simulink model "Twotanks_Model_TCGen"  (R2017b)
settings: Solver=FixedStepAuto  StartTime=0.0  StopTime=simTime  FixedStep=0.1  RelTol=1e-3  EnableMultiTasking=on
model workspace (MAT data in the model file):
  F = [0; 0]
  Global = [3707764736; 2; 1; 1; 1; 1]
  InputSize = 5
  Operation = 'value'
  X = [1.91912110987  0.7189344389; 0.667300428728  0.319032887648; 0.539327875678  0.291550549769; 1.11428719774  0.782058235411; 0.458496889769  0.886118463221]
  cs : Simulink.ConfigSet (value not decoded)
  curPath = '/Users/ceren.gebizli/Desktop/Shiva/QRA-Search/QRA-Search/Problems/SimulinkTesting'
  ext = ''
  generatedFile = '/Users/khouloud.gaaloul/Documents/Projects/SOCRaTeS/socrates/software/scalability/Simulink_Models/Twotanks/Twotanks_Model'
  hws = [3707764736; 2; 1; 1; 1; 1]
  input = [1.91912110987  0.7189344389; 0.667300428728  0.319032887648; 0.539327875678  0.291550549769; 1.11428719774  0.782058235411; 0.458496889769  0.886118463221]
  inputSize = 1
  j = 2
  m = matlab.io.MatFile
  m.Properties = matlab.io.matfile.Properties
  m.Properties.SupportsPartialAccess = 0
  m.Properties.Source = '/Users/khouloud.gaaloul/Documents/Projects/SOCRaTeS/socrates/software/scalability/RQ3/testcases/twotanks_tc_1.mat'
  matfilename = 'twotanks_tc_1.mat'
  model_cs : Simulink.ConfigSet (value not decoded)
  modelpath = '/Users/khouloud.gaaloul/Documents/Projects/SOCRaTeS/socrates/software/scalability/Simulink_Models/Twotanks/'
  name = 'Twotanks_Model'
  nbrInputs = 2
  nbrTimeSteps = 5001
  p = 1
  path = '/Users/khouloud.gaaloul/Documents/Projects/SOCRaTeS/socrates/software/scalability/Simulink_Models/Twotanks'
  pr.model_name = 'Twotanks_Model'
  pr.fc = 5000
  pr.stime = 500
  problem : class16 (value not decoded)
  problems = {'twotanks'}
  tank1_init_height_m = 1.91912110987
  tank2_init_height_m = 0.7189344389
  testcase.signal = [0.0460270741829 0.899426437102]
  timestep = 2
  var.signal = [0.0460270741829 0.899426437102]
values from neighbouring files (symbols this model uses):
  tank1_cross_section_area_m2_in = TC(i).tank1_cross_section_area_m2    [GetWhiteBoxData.m]    (also in MutationTesting.m; TCGeneration.m)
  tank1_pump_flow_rate_m3s_in = TC(i).tank1_pump_flow_rate_m3s    [GetWhiteBoxData.m]    (also in MutationTesting.m; TCGeneration.m)
  tank1_sensor_hi_height_m_in = TC(i).tank1_sensor_hi_height_m    [GetWhiteBoxData.m]    (also in MutationTesting.m; TCGeneration.m)
  tank1_sensor_lo_height_m_in = TC(i).tank1_sensor_lo_height_m    [GetWhiteBoxData.m]    (also in MutationTesting.m; TCGeneration.m)
  tank1_valve_flow_rate_m3s_in = TC(i).tank1_valve_flow_rate_m3s    [GetWhiteBoxData.m]    (also in MutationTesting.m; TCGeneration.m)
  tank2_cross_section_area_m2_in = TC(i).tank2_cross_section_area_m2    [GetWhiteBoxData.m]    (also in MutationTesting.m; TCGeneration.m)
  tank2_e_valve_flow_rate_m3s_in = TC(i).tank2_e_valve_flow_rate_m3s    [GetWhiteBoxData.m]    (also in MutationTesting.m; TCGeneration.m)
  tank2_p_valve_flow_rate_m3s_in = TC(i).tank2_p_valve_flow_rate_m3s    [GetWhiteBoxData.m]    (also in MutationTesting.m; TCGeneration.m)
  tank2_sensor_hi_height_m_in = TC(i).tank2_sensor_hi_height_m    [GetWhiteBoxData.m]    (also in MutationTesting.m; TCGeneration.m)
  tank2_sensor_lo_height_m_in = TC(i).tank2_sensor_lo_height_m    [GetWhiteBoxData.m]    (also in MutationTesting.m; TCGeneration.m)
  tank2_sensor_md_height_m_in = TC(i).tank2_sensor_md_height_m    [GetWhiteBoxData.m]    (also in MutationTesting.m; TCGeneration.m)
libraries: simulink x12
(part 1 of 2)
settings Model: Creator=Kerianne  LastModifiedBy=ainhoa.arruabarrena
settings DataIOCC: ExternalInput=var  LimitDataPoints=on  SaveFormat=StructureWithTime  SignalLoggingSaveFormat=ModelDataLogs  OutputSaveName=varout  LoggingToFile=on
settings OptimizationCC: DefaultParameterBehavior=Inlined  ExpressionDepthLimit=2147483647  LifeSpan=inf
settings DebuggingCC: UnderspecifiedInitializationDetection=Classic  MergeDetectMultiDrivingBlocksExec=none  SolverPrmCheckMsg=warning  MultiTaskDSMMsg=warning  MultiTaskCondExecSysMsg=none  StateNameClashWarn=warning  SFUnexpectedBacktrackingDiag=warning  SFNoUnconditionalDefaultTransitionDiag=warning  SFExecutionAtInitializationDiag=none
settings HardwareCC: ProdBitPerPointer=32  ProdBitPerSizeT=32  ProdBitPerPtrDiffT=32  ProdLargestAtomicFloat=None  ProdIntDivRoundTo=Undefined  ProdEndianess=Unspecified  ProdWordSize=32  ProdHWDeviceType=32-bit Generic
settings ModelReferenceCC: PropagateSignalLabelsOutOfModel=off
settings CodeAppCC: StateflowObjectComments=on
settings GRTTargetCC: TargetLangStandard=C89/C90 (ANSI)  GeneratePreprocessorConditionals=Disable all
settings ConfigComp: CovMetricSettings=dw  CovHtmlReporting=on  CovSaveCumulativeToWorkspaceVar=on  CovSaveSingleToWorkspaceVar=on  CovExternalEMLEnable=off

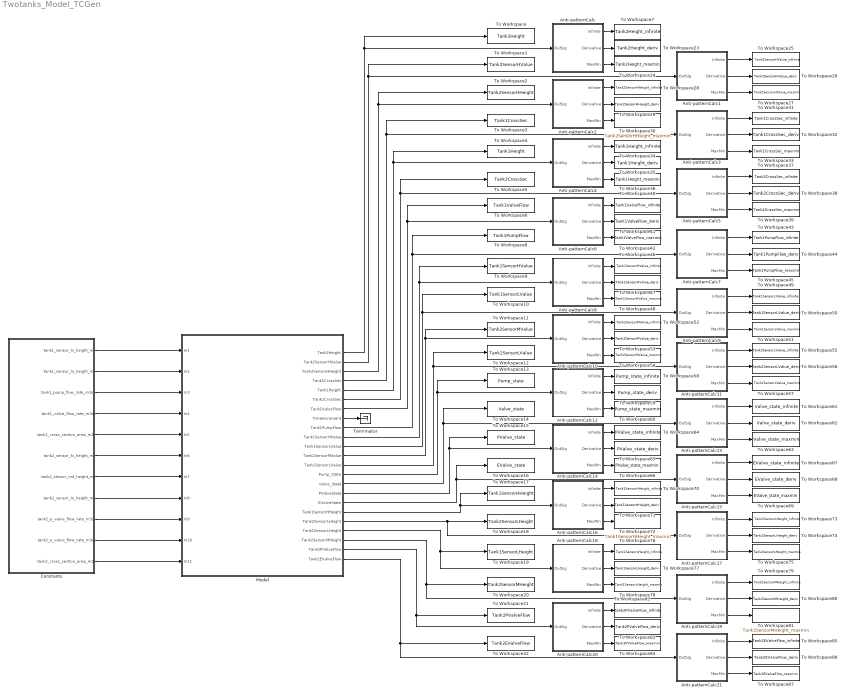
== system Twotanks_Model_TCGen ==
  Anti-patternCalc : Subsystem
  Anti-patternCalc1 : Subsystem
  Anti-patternCalc10 : Subsystem
  Anti-patternCalc11 : Subsystem
  Anti-patternCalc12 : Subsystem
  Anti-patternCalc13 : Subsystem
  Anti-patternCalc14 : Subsystem
  Anti-patternCalc15 : Subsystem
  Anti-patternCalc16 : Subsystem
  Anti-patternCalc17 : Subsystem
  Anti-patternCalc18 : Subsystem
  Anti-patternCalc19 : Subsystem
  Anti-patternCalc2 : Subsystem
  Anti-patternCalc20 : Subsystem
  Anti-patternCalc21 : Subsystem
  Anti-patternCalc3 : Subsystem
  Anti-patternCalc4 : Subsystem
  Anti-patternCalc5 : Subsystem
  Anti-patternCalc6 : Subsystem
  Anti-patternCalc7 : Subsystem
  Anti-patternCalc8 : Subsystem
  Anti-patternCalc9 : Subsystem
  Constants : Subsystem
  Model : Subsystem
  Terminator : Terminator
  To Workspace : ToWorkspace  VariableName=Tank2Height  SampleTime=-1
  To Workspace1 : ToWorkspace  VariableName=Tank2SensorHValue  SampleTime=-1
  To Workspace10 : ToWorkspace  VariableName=Tank1SensorLValue  SampleTime=-1
  To Workspace11 : ToWorkspace  VariableName=Tank2SensorMValue  SampleTime=-1
  To Workspace12 : ToWorkspace  VariableName=Tank2SensorLValue  SampleTime=-1
  To Workspace13 : ToWorkspace  VariableName=Pump_state  SampleTime=-1
  To Workspace14 : ToWorkspace  VariableName=Valve_state  SampleTime=-1
  To Workspace15 : ToWorkspace  VariableName=PValve_state  SampleTime=-1
  To Workspace16 : ToWorkspace  VariableName=EValve_state  SampleTime=-1
  To Workspace17 : ToWorkspace  VariableName=Tank1SensorHHeight  SampleTime=-1
  To Workspace18 : ToWorkspace  VariableName=Tank2SensorLHeight  SampleTime=-1
  To Workspace19 : ToWorkspace  VariableName=Tank1SensorLHeight  SampleTime=-1
  To Workspace2 : ToWorkspace  VariableName=Tank2SensorHHeight  SampleTime=-1
  To Workspace20 : ToWorkspace  VariableName=Tank2SensorMHeight  SampleTime=-1
  To Workspace21 : ToWorkspace  VariableName=Tank2PValveFlow  SampleTime=-1
  To Workspace22 : ToWorkspace  VariableName=Tank2EValveFlow  SampleTime=-1
  To Workspace23 : ToWorkspace  VariableName=Tank2Height_deriv  SampleTime=-1
  To Workspace24 : ToWorkspace  VariableName=Tank2Height_maxmin  SampleTime=-1
  To Workspace25 : ToWorkspace  VariableName=Tank2SensorHValue_infinite  SampleTime=-1
  To Workspace26 : ToWorkspace  VariableName=Tank2SensorHValue_deriv  SampleTime=-1
  To Workspace27 : ToWorkspace  VariableName=Tank2SensorHValue_maxmin  SampleTime=-1
  To Workspace28 : ToWorkspace  VariableName=Tank2SensorHHeight_infinite  SampleTime=-1
  To Workspace29 : ToWorkspace  VariableName=Tank2SensorHHeight_deriv  SampleTime=-1
  To Workspace3 : ToWorkspace  VariableName=Tank1CrossSec  SampleTime=-1
  To Workspace30 : ToWorkspace  VariableName=Tank2SensorHHeight_maxmin  SampleTime=-1
  To Workspace31 : ToWorkspace  VariableName=Tank1CrossSec_infinite  SampleTime=-1
  To Workspace32 : ToWorkspace  VariableName=Tank1CrossSec_deriv  SampleTime=-1
  To Workspace33 : ToWorkspace  VariableName=Tank1CrossSec_maxmin  SampleTime=-1
  To Workspace34 : ToWorkspace  VariableName=Tank1Height_infinite  SampleTime=-1
  To Workspace35 : ToWorkspace  VariableName=Tank1Height_deriv  SampleTime=-1
  To Workspace36 : ToWorkspace  VariableName=Tank1Height_maxmin  SampleTime=-1
  To Workspace37 : ToWorkspace  VariableName=Tank2CrossSec_infinite  SampleTime=-1
  To Workspace38 : ToWorkspace  VariableName=Tank2CrossSec_deriv  SampleTime=-1
  To Workspace39 : ToWorkspace  VariableName=Tank2CrossSec_maxmin  SampleTime=-1
  To Workspace4 : ToWorkspace  VariableName=Tank1Height  SampleTime=-1
  To Workspace40 : ToWorkspace  VariableName=Tank1ValveFlow_infinite  SampleTime=-1
  To Workspace41 : ToWorkspace  VariableName=Tank1ValveFlow_deriv  SampleTime=-1
  To Workspace42 : ToWorkspace  VariableName=Tank1ValveFlow_maxmin  SampleTime=-1
  To Workspace43 : ToWorkspace  VariableName=Tank1PumpFlow_infinite  SampleTime=-1
  To Workspace44 : ToWorkspace  VariableName=Tank1PumpFlow_deriv  SampleTime=-1
  To Workspace45 : ToWorkspace  VariableName=Tank1PumpFlow_maxmin  SampleTime=-1
  To Workspace46 : ToWorkspace  VariableName=Tank1SensorHValue_infinite  SampleTime=-1
  To Workspace47 : ToWorkspace  VariableName=Tank1SensorHValue_deriv  SampleTime=-1
  To Workspace48 : ToWorkspace  VariableName=Tank1SensorHValue_maxmin  SampleTime=-1
  To Workspace49 : ToWorkspace  VariableName=Tank1SensorLValue_infinite  SampleTime=-1
  To Workspace5 : ToWorkspace  VariableName=Tank2CrossSec  SampleTime=-1
  To Workspace50 : ToWorkspace  VariableName=Tank1SensorLValue_deriv  SampleTime=-1
  To Workspace51 : ToWorkspace  VariableName=Tank1SensorLValue_maxmin  SampleTime=-1
  To Workspace52 : ToWorkspace  VariableName=Tank2SensorMValue_infinite  SampleTime=-1
  To Workspace53 : ToWorkspace  VariableName=Tank2SensorMValue_deriv  SampleTime=-1
  To Workspace54 : ToWorkspace  VariableName=Tank2SensorMValue_maxmin  SampleTime=-1
  To Workspace55 : ToWorkspace  VariableName=Tank2SensorLValue_infinite  SampleTime=-1
  To Workspace56 : ToWorkspace  VariableName=Tank2SensorLValue_deriv  SampleTime=-1
  To Workspace57 : ToWorkspace  VariableName=Tank2SensorLValue_maxmin  SampleTime=-1
  To Workspace58 : ToWorkspace  VariableName=Pump_state_infinite  SampleTime=-1
  To Workspace59 : ToWorkspace  VariableName=Pump_state_deriv  SampleTime=-1
  To Workspace6 : ToWorkspace  VariableName=Tank1ValveFlow  SampleTime=-1
  To Workspace60 : ToWorkspace  VariableName=Pump_state_maxmin  SampleTime=-1
  To Workspace61 : ToWorkspace  VariableName=Valve_state_infinite  SampleTime=-1
  To Workspace62 : ToWorkspace  VariableName=Valve_state_deriv  SampleTime=-1
  To Workspace63 : ToWorkspace  VariableName=Valve_state_maxmin  SampleTime=-1
  To Workspace64 : ToWorkspace  VariableName=PValve_state_infinite  SampleTime=-1
  To Workspace65 : ToWorkspace  VariableName=PValve_state_deriv  SampleTime=-1
  To Workspace66 : ToWorkspace  VariableName=PValve_state_maxmin  SampleTime=-1
  To Workspace67 : ToWorkspace  VariableName=EValve_state_infinite  SampleTime=-1
  To Workspace68 : ToWorkspace  VariableName=EValve_state_deriv  SampleTime=-1
  To Workspace69 : ToWorkspace  VariableName=EValve_state_maxmin  SampleTime=-1
  To Workspace7 : ToWorkspace  VariableName=Tank2Height_infinite  SampleTime=-1
  To Workspace70 : ToWorkspace  VariableName=Tank1SensorHHeight_infinite  SampleTime=-1
  To Workspace71 : ToWorkspace  VariableName=Tank1SensorHHeight_deriv  SampleTime=-1
  To Workspace72 : ToWorkspace  VariableName=Tank1SensorHHeight_maxmin  SampleTime=-1
  To Workspace73 : ToWorkspace  VariableName=Tank2SensorLHeight_infinite  SampleTime=-1
  To Workspace74 : ToWorkspace  VariableName=Tank2SensorLHeight_deriv  SampleTime=-1
  To Workspace75 : ToWorkspace  VariableName=Tank2SensorLHeight_maxmin  SampleTime=-1
  To Workspace76 : ToWorkspace  VariableName=Tank1SensorLHeight_infinite  SampleTime=-1
  To Workspace77 : ToWorkspace  VariableName=Tank1SensorLHeight_deriv  SampleTime=-1
  To Workspace78 : ToWorkspace  VariableName=Tank1SensorLHeight_maxmin  SampleTime=-1
  To Workspace79 : ToWorkspace  VariableName=Tank2SensorMHeight_infinite  SampleTime=-1
  To Workspace8 : ToWorkspace  VariableName=Tank1PumpFlow  SampleTime=-1
  To Workspace80 : ToWorkspace  VariableName=Tank2SensorMHeight_deriv  SampleTime=-1
  To Workspace81 : ToWorkspace  VariableName=Tank2SensorMHeight_maxmin  SampleTime=-1
  To Workspace82 : ToWorkspace  VariableName=Tank2PValveFlow_infinite  SampleTime=-1
  To Workspace83 : ToWorkspace  VariableName=Tank2PValveFlow_deriv  SampleTime=-1
  To Workspace84 : ToWorkspace  VariableName=Tank2PValveFlow_maxmin  SampleTime=-1
  To Workspace85 : ToWorkspace  VariableName=Tank2EValveFlow_infinite  SampleTime=-1
  To Workspace86 : ToWorkspace  VariableName=Tank2EValveFlow_deriv  SampleTime=-1
  To Workspace87 : ToWorkspace  VariableName=Tank2EValveFlow_maxmin  SampleTime=-1
  To Workspace9 : ToWorkspace  VariableName=Tank1SensorHValue  SampleTime=-1
  wires:
  Constants/1(tank1_sensor_hi_height_m) -> Model/1(In1)
  Constants/2(tank1_sensor_lo_height_m) -> Model/2(In2)
  Constants/3(tank1_pump_flow_rate_m3s) -> Model/3(In3)
  Constants/4(tank1_valve_flow_rate_m3s) -> Model/4(In4)
  Constants/5(tank1_cross_section_area_m2) -> Model/5(In5)
  Constants/6(tank2_sensor_hi_height_m) -> Model/6(In6)
  Constants/7(tank2_sensor_md_height_m) -> Model/7(In7)
  Constants/8(tank2_sensor_lo_height_m) -> Model/8(In8)
  Constants/9(tank2_p_valve_flow_rate_m3s) -> Model/9(In9)
  Constants/10(tank2_e_valve_flow_rate_m3s) -> Model/10(In10)
  Constants/11(tank2_cross_section_area_m2) -> Model/11(In11)
  Model/1(Tank2Height) -> To Workspace/1, Anti-patternCalc/1(OutSig)
  Model/2(Tank2SensorHValue) -> Anti-patternCalc1/1(OutSig), To Workspace1/1
  Model/3(Tank2SensorHHeight) -> Anti-patternCalc2/1(OutSig), To Workspace2/1
  Model/7(Tank1ValveFlow) -> Anti-patternCalc6/1(OutSig), To Workspace6/1
  Model/8(TimeIncrement) -> Terminator/1
  Model/6(Tank2CrossSec) -> Anti-patternCalc5/1(OutSig), To Workspace5/1
  Model/5(Tank1Height) -> Anti-patternCalc4/1(OutSig), To Workspace4/1
  Model/9(Tank1PumpFlow) -> To Workspace8/1, Anti-patternCalc7/1(OutSig)
  Model/10(Tank1SensorHValue) -> Anti-patternCalc8/1(OutSig), To Workspace9/1
  Model/11(Tank1SensorLValue) -> To Workspace10/1, Anti-patternCalc9/1(OutSig)
  Model/12(Tank2SensorMValue) -> To Workspace11/1, Anti-patternCalc10/1(OutSig)
  Model/13(Tank2SensorLValue) -> Anti-patternCalc11/1(OutSig), To Workspace12/1
  Model/16(PValveState) -> Anti-patternCalc14/1(OutSig), To Workspace15/1
  Model/15(Valve_State) -> Anti-patternCalc13/1(OutSig), To Workspace14/1
  Model/14(Pump_State) -> Anti-patternCalc12/1(OutSig), To Workspace13/1
  Model/19(Tank2SensorLHeight) -> Anti-patternCalc17/1(OutSig), To Workspace18/1
  Model/18(Tank1SensorHHeight) -> Anti-patternCalc16/1(OutSig), To Workspace17/1
  Model/17(EValveState) -> Anti-patternCalc15/1(OutSig), To Workspace16/1
  Model/20(Tank1SensorLHeight) -> Anti-patternCalc18/1(OutSig), To Workspace19/1
  Model/21(Tank2SensorMHeight) -> To Workspace20/1, Anti-patternCalc19/1(OutSig)
  Model/23(Tank2EValveFlow) -> Anti-patternCalc21/1(OutSig), To Workspace22/1
  Model/22(Tank2PValveFlow) -> Anti-patternCalc20/1(OutSig), To Workspace21/1
  Anti-patternCalc/1(Infinite) -> To Workspace7/1
  Anti-patternCalc/2(Derivative) -> To Workspace23/1
  Anti-patternCalc/3(MaxMin) -> To Workspace24/1
  Anti-patternCalc1/1(Infinite) -> To Workspace25/1
  Anti-patternCalc1/3(MaxMin) -> To Workspace27/1
  Anti-patternCalc1/2(Derivative) -> To Workspace26/1
  Anti-patternCalc2/1(Infinite) -> To Workspace28/1
  Anti-patternCalc2/2(Derivative) -> To Workspace29/1
  Anti-patternCalc2/3(MaxMin) -> To Workspace30/1
  Model/4(Tank1CrossSec) -> Anti-patternCalc3/1(OutSig), To Workspace3/1
  Anti-patternCalc3/3(MaxMin) -> To Workspace33/1
  Anti-patternCalc3/2(Derivative) -> To Workspace32/1
  Anti-patternCalc3/1(Infinite) -> To Workspace31/1
  Anti-patternCalc4/1(Infinite) -> To Workspace34/1
  Anti-patternCalc4/2(Derivative) -> To Workspace35/1
  Anti-patternCalc4/3(MaxMin) -> To Workspace36/1
  Anti-patternCalc5/3(MaxMin) -> To Workspace39/1
  Anti-patternCalc5/2(Derivative) -> To Workspace38/1
  Anti-patternCalc5/1(Infinite) -> To Workspace37/1
  Anti-patternCalc6/1(Infinite) -> To Workspace40/1
  Anti-patternCalc6/2(Derivative) -> To Workspace41/1
  Anti-patternCalc6/3(MaxMin) -> To Workspace42/1
  Anti-patternCalc7/1(Infinite) -> To Workspace43/1
  Anti-patternCalc7/3(MaxMin) -> To Workspace45/1
  Anti-patternCalc7/2(Derivative) -> To Workspace44/1
  Anti-patternCalc8/1(Infinite) -> To Workspace46/1
  Anti-patternCalc8/2(Derivative) -> To Workspace47/1
  Anti-patternCalc8/3(MaxMin) -> To Workspace48/1
  Anti-patternCalc9/1(Infinite) -> To Workspace49/1
  Anti-patternCalc9/2(Derivative) -> To Workspace50/1
  Anti-patternCalc9/3(MaxMin) -> To Workspace51/1
  Anti-patternCalc10/1(Infinite) -> To Workspace52/1
  Anti-patternCalc10/2(Derivative) -> To Workspace53/1
  Anti-patternCalc10/3(MaxMin) -> To Workspace54/1
  Anti-patternCalc11/3(MaxMin) -> To Workspace57/1
  Anti-patternCalc11/2(Derivative) -> To Workspace56/1
  Anti-patternCalc11/1(Infinite) -> To Workspace55/1
  Anti-patternCalc12/1(Infinite) -> To Workspace58/1
  Anti-patternCalc12/2(Derivative) -> To Workspace59/1
  Anti-patternCalc12/3(MaxMin) -> To Workspace60/1
  Anti-patternCalc13/1(Infinite) -> To Workspace61/1
  Anti-patternCalc13/2(Derivative) -> To Workspace62/1
  Anti-patternCalc13/3(MaxMin) -> To Workspace63/1
  Anti-patternCalc14/1(Infinite) -> To Workspace64/1
  Anti-patternCalc14/2(Derivative) -> To Workspace65/1
  Anti-patternCalc14/3(MaxMin) -> To Workspace66/1
  Anti-patternCalc15/3(MaxMin) -> To Workspace69/1
  Anti-patternCalc15/2(Derivative) -> To Workspace68/1
  Anti-patternCalc15/1(Infinite) -> To Workspace67/1
  Anti-patternCalc16/1(Infinite) -> To Workspace70/1
  Anti-patternCalc16/2(Derivative) -> To Workspace71/1
  Anti-patternCalc16/3(MaxMin) -> To Workspace72/1
  Anti-patternCalc17/1(Infinite) -> To Workspace73/1
  Anti-patternCalc17/2(Derivative) -> To Workspace74/1
  Anti-patternCalc17/3(MaxMin) -> To Workspace75/1
  Anti-patternCalc18/1(Infinite) -> To Workspace76/1
  Anti-patternCalc18/2(Derivative) -> To Workspace77/1
  Anti-patternCalc18/3(MaxMin) -> To Workspace78/1
  Anti-patternCalc19/1(Infinite) -> To Workspace79/1
  Anti-patternCalc19/3(MaxMin) -> To Workspace81/1
  Anti-patternCalc19/2(Derivative) -> To Workspace80/1
  Anti-patternCalc20/1(Infinite) -> To Workspace82/1
  Anti-patternCalc20/2(Derivative) -> To Workspace83/1
  Anti-patternCalc20/3(MaxMin) -> To Workspace84/1
  Anti-patternCalc21/1(Infinite) -> To Workspace85/1
  Anti-patternCalc21/2(Derivative) -> To Workspace86/1
  Anti-patternCalc21/3(MaxMin) -> To Workspace87/1

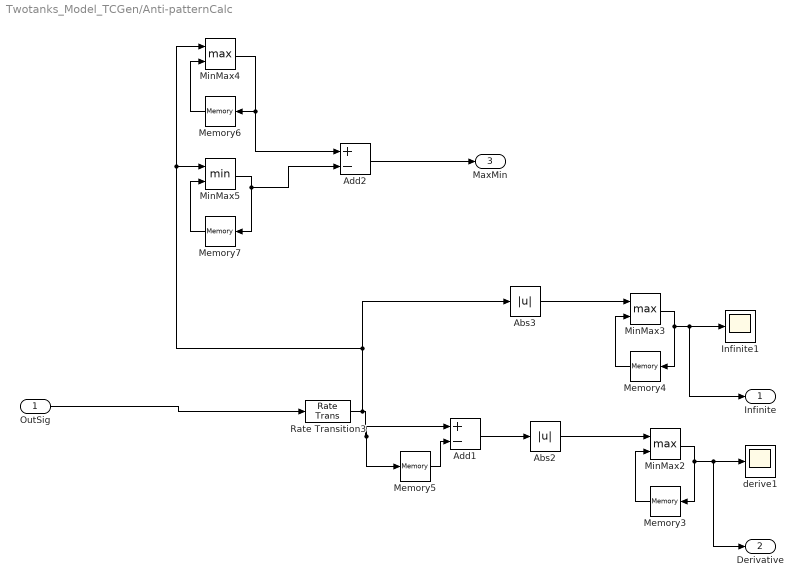
== system Twotanks_Model_TCGen/Anti-patternCalc ==
  OutSig : Inport
  Abs2 : Abs
  Abs3 : Abs
  Add1 : Sum  Inputs=+-
  Add2 : Sum  Inputs=+-
  Infinite1 : Scope
  Memory{3..7} (5 alike) : Memory
  MinMax2 : MinMax  Function=max  Inputs=2
  MinMax3 : MinMax  Function=max  Inputs=2
  MinMax4 : MinMax  Function=max  Inputs=2
  MinMax5 : MinMax  Inputs=2
  Rate Transition3 : RateTransition
  derive1 : Scope
  Infinite : Outport
  Derivative : Outport  Port=2
  MaxMin : Outport  Port=3
  wires:
  MinMax5/1 -> Add2/2, Memory7/1
  Abs2/1 -> MinMax2/1
  Memory4/1 -> MinMax3/2
  Memory3/1 -> MinMax2/2
  MinMax4/1 -> Add2/1, Memory6/1
  Memory7/1 -> MinMax5/2
  Add1/1 -> Abs2/1
  Memory6/1 -> MinMax4/2
  Memory5/1 -> Add1/2
  Rate Transition3/1 -> MinMax4/1, MinMax5/1, Abs3/1, Add1/1, Memory5/1
  Abs3/1 -> MinMax3/1
  MinMax2/1 -> Derivative/1, derive1/1, Memory3/1
  OutSig/1 -> Rate Transition3/1
  MinMax3/1 -> Memory4/1, Infinite/1, Infinite1/1
  Add2/1 -> MaxMin/1

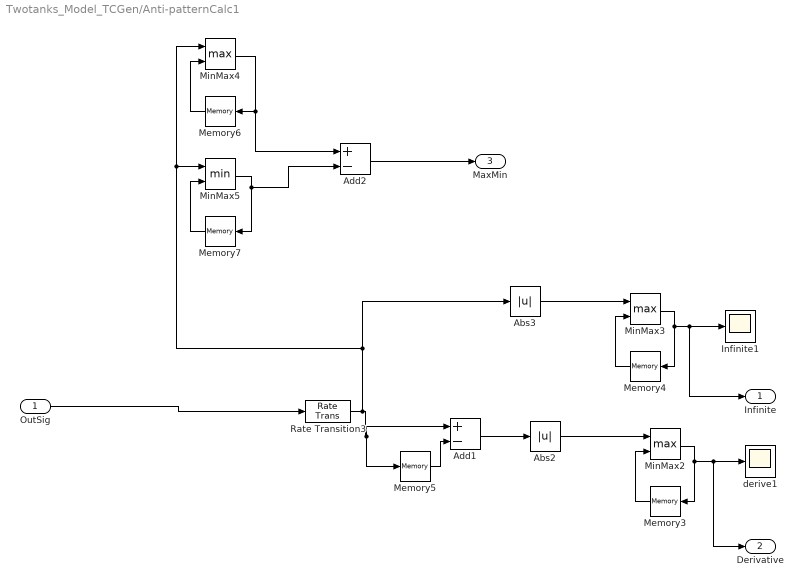
== system Twotanks_Model_TCGen/Anti-patternCalc1 ==
  OutSig : Inport
  Abs2 : Abs
  Abs3 : Abs
  Add1 : Sum  Inputs=+-
  Add2 : Sum  Inputs=+-
  Infinite1 : Scope
  Memory{3..7} (5 alike) : Memory
  MinMax2 : MinMax  Function=max  Inputs=2
  MinMax3 : MinMax  Function=max  Inputs=2
  MinMax4 : MinMax  Function=max  Inputs=2
  MinMax5 : MinMax  Inputs=2
  Rate Transition3 : RateTransition
  derive1 : Scope
  Infinite : Outport
  Derivative : Outport  Port=2
  MaxMin : Outport  Port=3
  wires:
  Add2/1 -> MaxMin/1
  MinMax3/1 -> Infinite1/1, Infinite/1, Memory4/1
  OutSig/1 -> Rate Transition3/1
  MinMax2/1 -> Memory3/1, derive1/1, Derivative/1
  Abs3/1 -> MinMax3/1
  Rate Transition3/1 -> Memory5/1, Add1/1, Abs3/1, MinMax5/1, MinMax4/1
  Memory5/1 -> Add1/2
  Memory6/1 -> MinMax4/2
  Add1/1 -> Abs2/1
  Memory7/1 -> MinMax5/2
  MinMax4/1 -> Memory6/1, Add2/1
  Memory3/1 -> MinMax2/2
  Memory4/1 -> MinMax3/2
  Abs2/1 -> MinMax2/1
  MinMax5/1 -> Memory7/1, Add2/2

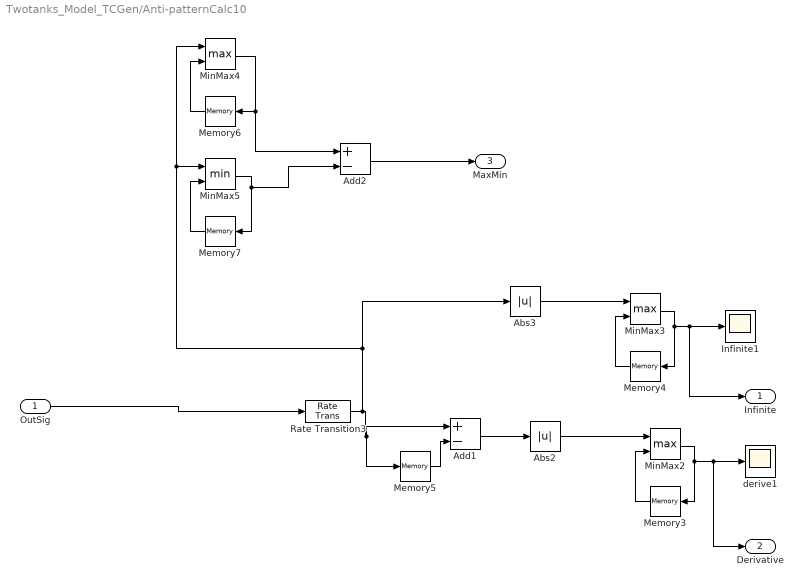
== system Twotanks_Model_TCGen/Anti-patternCalc10 ==
  OutSig : Inport
  Abs2 : Abs
  Abs3 : Abs
  Add1 : Sum  Inputs=+-
  Add2 : Sum  Inputs=+-
  Infinite1 : Scope
  Memory{3..7} (5 alike) : Memory
  MinMax2 : MinMax  Function=max  Inputs=2
  MinMax3 : MinMax  Function=max  Inputs=2
  MinMax4 : MinMax  Function=max  Inputs=2
  MinMax5 : MinMax  Inputs=2
  Rate Transition3 : RateTransition
  derive1 : Scope
  Infinite : Outport
  Derivative : Outport  Port=2
  MaxMin : Outport  Port=3
  wires:
  Add2/1 -> MaxMin/1
  MinMax3/1 -> Infinite1/1, Infinite/1, Memory4/1
  OutSig/1 -> Rate Transition3/1
  MinMax2/1 -> Memory3/1, derive1/1, Derivative/1
  Abs3/1 -> MinMax3/1
  Rate Transition3/1 -> Memory5/1, Add1/1, Abs3/1, MinMax5/1, MinMax4/1
  Memory5/1 -> Add1/2
  Memory6/1 -> MinMax4/2
  Add1/1 -> Abs2/1
  Memory7/1 -> MinMax5/2
  MinMax4/1 -> Memory6/1, Add2/1
  Memory3/1 -> MinMax2/2
  Memory4/1 -> MinMax3/2
  Abs2/1 -> MinMax2/1
  MinMax5/1 -> Memory7/1, Add2/2

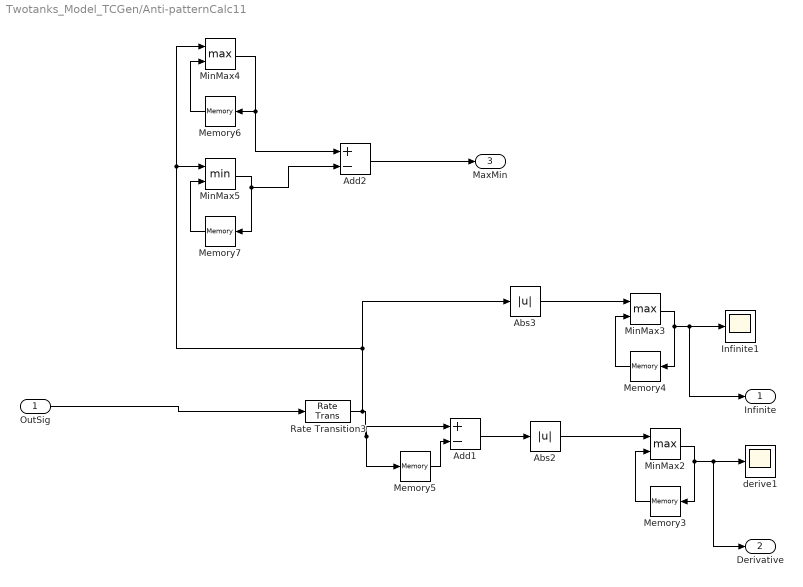
== system Twotanks_Model_TCGen/Anti-patternCalc11 ==
  OutSig : Inport
  Abs2 : Abs
  Abs3 : Abs
  Add1 : Sum  Inputs=+-
  Add2 : Sum  Inputs=+-
  Infinite1 : Scope
  Memory{3..7} (5 alike) : Memory
  MinMax2 : MinMax  Function=max  Inputs=2
  MinMax3 : MinMax  Function=max  Inputs=2
  MinMax4 : MinMax  Function=max  Inputs=2
  MinMax5 : MinMax  Inputs=2
  Rate Transition3 : RateTransition
  derive1 : Scope
  Infinite : Outport
  Derivative : Outport  Port=2
  MaxMin : Outport  Port=3
  wires:
  MinMax5/1 -> Add2/2, Memory7/1
  Abs2/1 -> MinMax2/1
  Memory4/1 -> MinMax3/2
  Memory3/1 -> MinMax2/2
  MinMax4/1 -> Add2/1, Memory6/1
  Memory7/1 -> MinMax5/2
  Add1/1 -> Abs2/1
  Memory6/1 -> MinMax4/2
  Memory5/1 -> Add1/2
  Rate Transition3/1 -> MinMax4/1, MinMax5/1, Abs3/1, Add1/1, Memory5/1
  Abs3/1 -> MinMax3/1
  MinMax2/1 -> Derivative/1, derive1/1, Memory3/1
  OutSig/1 -> Rate Transition3/1
  MinMax3/1 -> Memory4/1, Infinite/1, Infinite1/1
  Add2/1 -> MaxMin/1

== system Twotanks_Model_TCGen/Anti-patternCalc12 ==
  OutSig : Inport
  Abs2 : Abs
  Abs3 : Abs
  Add1 : Sum  Inputs=+-
  Add2 : Sum  Inputs=+-
  Infinite1 : Scope
  Memory{3..7} (5 alike) : Memory
  MinMax2 : MinMax  Function=max  Inputs=2
  MinMax3 : MinMax  Function=max  Inputs=2
  MinMax4 : MinMax  Function=max  Inputs=2
  MinMax5 : MinMax  Inputs=2
  Rate Transition3 : RateTransition
  derive1 : Scope
  Infinite : Outport
  Derivative : Outport  Port=2
  MaxMin : Outport  Port=3
  wires:
  MinMax5/1 -> Add2/2, Memory7/1
  Abs2/1 -> MinMax2/1
  Memory4/1 -> MinMax3/2
  Memory3/1 -> MinMax2/2
  MinMax4/1 -> Add2/1, Memory6/1
  Memory7/1 -> MinMax5/2
  Add1/1 -> Abs2/1
  Memory6/1 -> MinMax4/2
  Memory5/1 -> Add1/2
  Rate Transition3/1 -> MinMax4/1, MinMax5/1, Abs3/1, Add1/1, Memory5/1
  Abs3/1 -> MinMax3/1
  MinMax2/1 -> Derivative/1, derive1/1, Memory3/1
  OutSig/1 -> Rate Transition3/1
  MinMax3/1 -> Memory4/1, Infinite/1, Infinite1/1
  Add2/1 -> MaxMin/1

== system Twotanks_Model_TCGen/Anti-patternCalc13 ==
  OutSig : Inport
  Abs2 : Abs
  Abs3 : Abs
  Add1 : Sum  Inputs=+-
  Add2 : Sum  Inputs=+-
  Infinite1 : Scope
  Memory{3..7} (5 alike) : Memory
  MinMax2 : MinMax  Function=max  Inputs=2
  MinMax3 : MinMax  Function=max  Inputs=2
  MinMax4 : MinMax  Function=max  Inputs=2
  MinMax5 : MinMax  Inputs=2
  Rate Transition3 : RateTransition
  derive1 : Scope
  Infinite : Outport
  Derivative : Outport  Port=2
  MaxMin : Outport  Port=3
  wires:
  Add2/1 -> MaxMin/1
  MinMax3/1 -> Infinite1/1, Infinite/1, Memory4/1
  OutSig/1 -> Rate Transition3/1
  MinMax2/1 -> Memory3/1, derive1/1, Derivative/1
  Abs3/1 -> MinMax3/1
  Rate Transition3/1 -> Memory5/1, Add1/1, Abs3/1, MinMax5/1, MinMax4/1
  Memory5/1 -> Add1/2
  Memory6/1 -> MinMax4/2
  Add1/1 -> Abs2/1
  Memory7/1 -> MinMax5/2
  MinMax4/1 -> Memory6/1, Add2/1
  Memory3/1 -> MinMax2/2
  Memory4/1 -> MinMax3/2
  Abs2/1 -> MinMax2/1
  MinMax5/1 -> Memory7/1, Add2/2

== system Twotanks_Model_TCGen/Anti-patternCalc14 ==
  OutSig : Inport
  Abs2 : Abs
  Abs3 : Abs
  Add1 : Sum  Inputs=+-
  Add2 : Sum  Inputs=+-
  Infinite1 : Scope
  Memory{3..7} (5 alike) : Memory
  MinMax2 : MinMax  Function=max  Inputs=2
  MinMax3 : MinMax  Function=max  Inputs=2
  MinMax4 : MinMax  Function=max  Inputs=2
  MinMax5 : MinMax  Inputs=2
  Rate Transition3 : RateTransition
  derive1 : Scope
  Infinite : Outport
  Derivative : Outport  Port=2
  MaxMin : Outport  Port=3
  wires:
  Add2/1 -> MaxMin/1
  MinMax3/1 -> Infinite1/1, Infinite/1, Memory4/1
  OutSig/1 -> Rate Transition3/1
  MinMax2/1 -> Memory3/1, derive1/1, Derivative/1
  Abs3/1 -> MinMax3/1
  Rate Transition3/1 -> Memory5/1, Add1/1, Abs3/1, MinMax5/1, MinMax4/1
  Memory5/1 -> Add1/2
  Memory6/1 -> MinMax4/2
  Add1/1 -> Abs2/1
  Memory7/1 -> MinMax5/2
  MinMax4/1 -> Memory6/1, Add2/1
  Memory3/1 -> MinMax2/2
  Memory4/1 -> MinMax3/2
  Abs2/1 -> MinMax2/1
  MinMax5/1 -> Memory7/1, Add2/2

== system Twotanks_Model_TCGen/Anti-patternCalc15 ==
  OutSig : Inport
  Abs2 : Abs
  Abs3 : Abs
  Add1 : Sum  Inputs=+-
  Add2 : Sum  Inputs=+-
  Infinite1 : Scope
  Memory{3..7} (5 alike) : Memory
  MinMax2 : MinMax  Function=max  Inputs=2
  MinMax3 : MinMax  Function=max  Inputs=2
  MinMax4 : MinMax  Function=max  Inputs=2
  MinMax5 : MinMax  Inputs=2
  Rate Transition3 : RateTransition
  derive1 : Scope
  Infinite : Outport
  Derivative : Outport  Port=2
  MaxMin : Outport  Port=3
  wires:
  MinMax5/1 -> Add2/2, Memory7/1
  Abs2/1 -> MinMax2/1
  Memory4/1 -> MinMax3/2
  Memory3/1 -> MinMax2/2
  MinMax4/1 -> Add2/1, Memory6/1
  Memory7/1 -> MinMax5/2
  Add1/1 -> Abs2/1
  Memory6/1 -> MinMax4/2
  Memory5/1 -> Add1/2
  Rate Transition3/1 -> MinMax4/1, MinMax5/1, Abs3/1, Add1/1, Memory5/1
  Abs3/1 -> MinMax3/1
  MinMax2/1 -> Derivative/1, derive1/1, Memory3/1
  OutSig/1 -> Rate Transition3/1
  MinMax3/1 -> Memory4/1, Infinite/1, Infinite1/1
  Add2/1 -> MaxMin/1

== system Twotanks_Model_TCGen/Anti-patternCalc16 ==
  OutSig : Inport
  Abs2 : Abs
  Abs3 : Abs
  Add1 : Sum  Inputs=+-
  Add2 : Sum  Inputs=+-
  Infinite1 : Scope
  Memory{3..7} (5 alike) : Memory
  MinMax2 : MinMax  Function=max  Inputs=2
  MinMax3 : MinMax  Function=max  Inputs=2
  MinMax4 : MinMax  Function=max  Inputs=2
  MinMax5 : MinMax  Inputs=2
  Rate Transition3 : RateTransition
  derive1 : Scope
  Infinite : Outport
  Derivative : Outport  Port=2
  MaxMin : Outport  Port=3
  wires:
  MinMax5/1 -> Add2/2, Memory7/1
  Abs2/1 -> MinMax2/1
  Memory4/1 -> MinMax3/2
  Memory3/1 -> MinMax2/2
  MinMax4/1 -> Add2/1, Memory6/1
  Memory7/1 -> MinMax5/2
  Add1/1 -> Abs2/1
  Memory6/1 -> MinMax4/2
  Memory5/1 -> Add1/2
  Rate Transition3/1 -> MinMax4/1, MinMax5/1, Abs3/1, Add1/1, Memory5/1
  Abs3/1 -> MinMax3/1
  MinMax2/1 -> Derivative/1, derive1/1, Memory3/1
  OutSig/1 -> Rate Transition3/1
  MinMax3/1 -> Memory4/1, Infinite/1, Infinite1/1
  Add2/1 -> MaxMin/1

== system Twotanks_Model_TCGen/Anti-patternCalc17 ==
  OutSig : Inport
  Abs2 : Abs
  Abs3 : Abs
  Add1 : Sum  Inputs=+-
  Add2 : Sum  Inputs=+-
  Infinite1 : Scope
  Memory{3..7} (5 alike) : Memory
  MinMax2 : MinMax  Function=max  Inputs=2
  MinMax3 : MinMax  Function=max  Inputs=2
  MinMax4 : MinMax  Function=max  Inputs=2
  MinMax5 : MinMax  Inputs=2
  Rate Transition3 : RateTransition
  derive1 : Scope
  Infinite : Outport
  Derivative : Outport  Port=2
  MaxMin : Outport  Port=3
  wires:
  Add2/1 -> MaxMin/1
  MinMax3/1 -> Infinite1/1, Infinite/1, Memory4/1
  OutSig/1 -> Rate Transition3/1
  MinMax2/1 -> Memory3/1, derive1/1, Derivative/1
  Abs3/1 -> MinMax3/1
  Rate Transition3/1 -> Memory5/1, Add1/1, Abs3/1, MinMax5/1, MinMax4/1
  Memory5/1 -> Add1/2
  Memory6/1 -> MinMax4/2
  Add1/1 -> Abs2/1
  Memory7/1 -> MinMax5/2
  MinMax4/1 -> Memory6/1, Add2/1
  Memory3/1 -> MinMax2/2
  Memory4/1 -> MinMax3/2
  Abs2/1 -> MinMax2/1
  MinMax5/1 -> Memory7/1, Add2/2

== system Twotanks_Model_TCGen/Anti-patternCalc18 ==
  OutSig : Inport
  Abs2 : Abs
  Abs3 : Abs
  Add1 : Sum  Inputs=+-
  Add2 : Sum  Inputs=+-
  Infinite1 : Scope
  Memory{3..7} (5 alike) : Memory
  MinMax2 : MinMax  Function=max  Inputs=2
  MinMax3 : MinMax  Function=max  Inputs=2
  MinMax4 : MinMax  Function=max  Inputs=2
  MinMax5 : MinMax  Inputs=2
  Rate Transition3 : RateTransition
  derive1 : Scope
  Infinite : Outport
  Derivative : Outport  Port=2
  MaxMin : Outport  Port=3
  wires:
  Add2/1 -> MaxMin/1
  MinMax3/1 -> Infinite1/1, Infinite/1, Memory4/1
  OutSig/1 -> Rate Transition3/1
  MinMax2/1 -> Memory3/1, derive1/1, Derivative/1
  Abs3/1 -> MinMax3/1
  Rate Transition3/1 -> Memory5/1, Add1/1, Abs3/1, MinMax5/1, MinMax4/1
  Memory5/1 -> Add1/2
  Memory6/1 -> MinMax4/2
  Add1/1 -> Abs2/1
  Memory7/1 -> MinMax5/2
  MinMax4/1 -> Memory6/1, Add2/1
  Memory3/1 -> MinMax2/2
  Memory4/1 -> MinMax3/2
  Abs2/1 -> MinMax2/1
  MinMax5/1 -> Memory7/1, Add2/2

== system Twotanks_Model_TCGen/Anti-patternCalc19 ==
  OutSig : Inport
  Abs2 : Abs
  Abs3 : Abs
  Add1 : Sum  Inputs=+-
  Add2 : Sum  Inputs=+-
  Infinite1 : Scope
  Memory{3..7} (5 alike) : Memory
  MinMax2 : MinMax  Function=max  Inputs=2
  MinMax3 : MinMax  Function=max  Inputs=2
  MinMax4 : MinMax  Function=max  Inputs=2
  MinMax5 : MinMax  Inputs=2
  Rate Transition3 : RateTransition
  derive1 : Scope
  Infinite : Outport
  Derivative : Outport  Port=2
  MaxMin : Outport  Port=3
  wires:
  MinMax5/1 -> Add2/2, Memory7/1
  Abs2/1 -> MinMax2/1
  Memory4/1 -> MinMax3/2
  Memory3/1 -> MinMax2/2
  MinMax4/1 -> Add2/1, Memory6/1
  Memory7/1 -> MinMax5/2
  Add1/1 -> Abs2/1
  Memory6/1 -> MinMax4/2
  Memory5/1 -> Add1/2
  Rate Transition3/1 -> MinMax4/1, MinMax5/1, Abs3/1, Add1/1, Memory5/1
  Abs3/1 -> MinMax3/1
  MinMax2/1 -> Derivative/1, derive1/1, Memory3/1
  OutSig/1 -> Rate Transition3/1
  MinMax3/1 -> Memory4/1, Infinite/1, Infinite1/1
  Add2/1 -> MaxMin/1

== system Twotanks_Model_TCGen/Anti-patternCalc2 ==
  OutSig : Inport
  Abs2 : Abs
  Abs3 : Abs
  Add1 : Sum  Inputs=+-
  Add2 : Sum  Inputs=+-
  Infinite1 : Scope
  Memory{3..7} (5 alike) : Memory
  MinMax2 : MinMax  Function=max  Inputs=2
  MinMax3 : MinMax  Function=max  Inputs=2
  MinMax4 : MinMax  Function=max  Inputs=2
  MinMax5 : MinMax  Inputs=2
  Rate Transition3 : RateTransition
  derive1 : Scope
  Infinite : Outport
  Derivative : Outport  Port=2
  MaxMin : Outport  Port=3
  wires:
  MinMax5/1 -> Add2/2, Memory7/1
  Abs2/1 -> MinMax2/1
  Memory4/1 -> MinMax3/2
  Memory3/1 -> MinMax2/2
  MinMax4/1 -> Add2/1, Memory6/1
  Memory7/1 -> MinMax5/2
  Add1/1 -> Abs2/1
  Memory6/1 -> MinMax4/2
  Memory5/1 -> Add1/2
  Rate Transition3/1 -> MinMax4/1, MinMax5/1, Abs3/1, Add1/1, Memory5/1
  Abs3/1 -> MinMax3/1
  MinMax2/1 -> Derivative/1, derive1/1, Memory3/1
  OutSig/1 -> Rate Transition3/1
  MinMax3/1 -> Memory4/1, Infinite/1, Infinite1/1
  Add2/1 -> MaxMin/1

== system Twotanks_Model_TCGen/Anti-patternCalc20 ==
  OutSig : Inport
  Abs2 : Abs
  Abs3 : Abs
  Add1 : Sum  Inputs=+-
  Add2 : Sum  Inputs=+-
  Infinite1 : Scope
  Memory{3..7} (5 alike) : Memory
  MinMax2 : MinMax  Function=max  Inputs=2
  MinMax3 : MinMax  Function=max  Inputs=2
  MinMax4 : MinMax  Function=max  Inputs=2
  MinMax5 : MinMax  Inputs=2
  Rate Transition3 : RateTransition
  derive1 : Scope
  Infinite : Outport
  Derivative : Outport  Port=2
  MaxMin : Outport  Port=3
  wires:
  MinMax5/1 -> Add2/2, Memory7/1
  Abs2/1 -> MinMax2/1
  Memory4/1 -> MinMax3/2
  Memory3/1 -> MinMax2/2
  MinMax4/1 -> Add2/1, Memory6/1
  Memory7/1 -> MinMax5/2
  Add1/1 -> Abs2/1
  Memory6/1 -> MinMax4/2
  Memory5/1 -> Add1/2
  Rate Transition3/1 -> MinMax4/1, MinMax5/1, Abs3/1, Add1/1, Memory5/1
  Abs3/1 -> MinMax3/1
  MinMax2/1 -> Derivative/1, derive1/1, Memory3/1
  OutSig/1 -> Rate Transition3/1
  MinMax3/1 -> Memory4/1, Infinite/1, Infinite1/1
  Add2/1 -> MaxMin/1

== system Twotanks_Model_TCGen/Anti-patternCalc21 ==
  OutSig : Inport
  Abs2 : Abs
  Abs3 : Abs
  Add1 : Sum  Inputs=+-
  Add2 : Sum  Inputs=+-
  Infinite1 : Scope
  Memory{3..7} (5 alike) : Memory
  MinMax2 : MinMax  Function=max  Inputs=2
  MinMax3 : MinMax  Function=max  Inputs=2
  MinMax4 : MinMax  Function=max  Inputs=2
  MinMax5 : MinMax  Inputs=2
  Rate Transition3 : RateTransition
  derive1 : Scope
  Infinite : Outport
  Derivative : Outport  Port=2
  MaxMin : Outport  Port=3
  wires:
  Add2/1 -> MaxMin/1
  MinMax3/1 -> Infinite1/1, Infinite/1, Memory4/1
  OutSig/1 -> Rate Transition3/1
  MinMax2/1 -> Memory3/1, derive1/1, Derivative/1
  Abs3/1 -> MinMax3/1
  Rate Transition3/1 -> Memory5/1, Add1/1, Abs3/1, MinMax5/1, MinMax4/1
  Memory5/1 -> Add1/2
  Memory6/1 -> MinMax4/2
  Add1/1 -> Abs2/1
  Memory7/1 -> MinMax5/2
  MinMax4/1 -> Memory6/1, Add2/1
  Memory3/1 -> MinMax2/2
  Memory4/1 -> MinMax3/2
  Abs2/1 -> MinMax2/1
  MinMax5/1 -> Memory7/1, Add2/2

== system Twotanks_Model_TCGen/Anti-patternCalc3 ==
  OutSig : Inport
  Abs2 : Abs
  Abs3 : Abs
  Add1 : Sum  Inputs=+-
  Add2 : Sum  Inputs=+-
  Infinite1 : Scope
  Memory{3..7} (5 alike) : Memory
  MinMax2 : MinMax  Function=max  Inputs=2
  MinMax3 : MinMax  Function=max  Inputs=2
  MinMax4 : MinMax  Function=max  Inputs=2
  MinMax5 : MinMax  Inputs=2
  Rate Transition3 : RateTransition
  derive1 : Scope
  Infinite : Outport
  Derivative : Outport  Port=2
  MaxMin : Outport  Port=3
  wires:
  Add2/1 -> MaxMin/1
  MinMax3/1 -> Infinite1/1, Infinite/1, Memory4/1
  OutSig/1 -> Rate Transition3/1
  MinMax2/1 -> Memory3/1, derive1/1, Derivative/1
  Abs3/1 -> MinMax3/1
  Rate Transition3/1 -> Memory5/1, Add1/1, Abs3/1, MinMax5/1, MinMax4/1
  Memory5/1 -> Add1/2
  Memory6/1 -> MinMax4/2
  Add1/1 -> Abs2/1
  Memory7/1 -> MinMax5/2
  MinMax4/1 -> Memory6/1, Add2/1
  Memory3/1 -> MinMax2/2
  Memory4/1 -> MinMax3/2
  Abs2/1 -> MinMax2/1
  MinMax5/1 -> Memory7/1, Add2/2

== system Twotanks_Model_TCGen/Anti-patternCalc4 ==
  OutSig : Inport
  Abs2 : Abs
  Abs3 : Abs
  Add1 : Sum  Inputs=+-
  Add2 : Sum  Inputs=+-
  Infinite1 : Scope
  Memory{3..7} (5 alike) : Memory
  MinMax2 : MinMax  Function=max  Inputs=2
  MinMax3 : MinMax  Function=max  Inputs=2
  MinMax4 : MinMax  Function=max  Inputs=2
  MinMax5 : MinMax  Inputs=2
  Rate Transition3 : RateTransition
  derive1 : Scope
  Infinite : Outport
  Derivative : Outport  Port=2
  MaxMin : Outport  Port=3
  wires:
  MinMax5/1 -> Add2/2, Memory7/1
  Abs2/1 -> MinMax2/1
  Memory4/1 -> MinMax3/2
  Memory3/1 -> MinMax2/2
  MinMax4/1 -> Add2/1, Memory6/1
  Memory7/1 -> MinMax5/2
  Add1/1 -> Abs2/1
  Memory6/1 -> MinMax4/2
  Memory5/1 -> Add1/2
  Rate Transition3/1 -> MinMax4/1, MinMax5/1, Abs3/1, Add1/1, Memory5/1
  Abs3/1 -> MinMax3/1
  MinMax2/1 -> Derivative/1, derive1/1, Memory3/1
  OutSig/1 -> Rate Transition3/1
  MinMax3/1 -> Memory4/1, Infinite/1, Infinite1/1
  Add2/1 -> MaxMin/1

== system Twotanks_Model_TCGen/Anti-patternCalc5 ==
  OutSig : Inport
  Abs2 : Abs
  Abs3 : Abs
  Add1 : Sum  Inputs=+-
  Add2 : Sum  Inputs=+-
  Infinite1 : Scope
  Memory{3..7} (5 alike) : Memory
  MinMax2 : MinMax  Function=max  Inputs=2
  MinMax3 : MinMax  Function=max  Inputs=2
  MinMax4 : MinMax  Function=max  Inputs=2
  MinMax5 : MinMax  Inputs=2
  Rate Transition3 : RateTransition
  derive1 : Scope
  Infinite : Outport
  Derivative : Outport  Port=2
  MaxMin : Outport  Port=3
  wires:
  MinMax5/1 -> Add2/2, Memory7/1
  Abs2/1 -> MinMax2/1
  Memory4/1 -> MinMax3/2
  Memory3/1 -> MinMax2/2
  MinMax4/1 -> Add2/1, Memory6/1
  Memory7/1 -> MinMax5/2
  Add1/1 -> Abs2/1
  Memory6/1 -> MinMax4/2
  Memory5/1 -> Add1/2
  Rate Transition3/1 -> MinMax4/1, MinMax5/1, Abs3/1, Add1/1, Memory5/1
  Abs3/1 -> MinMax3/1
  MinMax2/1 -> Derivative/1, derive1/1, Memory3/1
  OutSig/1 -> Rate Transition3/1
  MinMax3/1 -> Memory4/1, Infinite/1, Infinite1/1
  Add2/1 -> MaxMin/1

== system Twotanks_Model_TCGen/Anti-patternCalc6 ==
  OutSig : Inport
  Abs2 : Abs
  Abs3 : Abs
  Add1 : Sum  Inputs=+-
  Add2 : Sum  Inputs=+-
  Infinite1 : Scope
  Memory{3..7} (5 alike) : Memory
  MinMax2 : MinMax  Function=max  Inputs=2
  MinMax3 : MinMax  Function=max  Inputs=2
  MinMax4 : MinMax  Function=max  Inputs=2
  MinMax5 : MinMax  Inputs=2
  Rate Transition3 : RateTransition
  derive1 : Scope
  Infinite : Outport
  Derivative : Outport  Port=2
  MaxMin : Outport  Port=3
  wires:
  Add2/1 -> MaxMin/1
  MinMax3/1 -> Infinite1/1, Infinite/1, Memory4/1
  OutSig/1 -> Rate Transition3/1
  MinMax2/1 -> Memory3/1, derive1/1, Derivative/1
  Abs3/1 -> MinMax3/1
  Rate Transition3/1 -> Memory5/1, Add1/1, Abs3/1, MinMax5/1, MinMax4/1
  Memory5/1 -> Add1/2
  Memory6/1 -> MinMax4/2
  Add1/1 -> Abs2/1
  Memory7/1 -> MinMax5/2
  MinMax4/1 -> Memory6/1, Add2/1
  Memory3/1 -> MinMax2/2
  Memory4/1 -> MinMax3/2
  Abs2/1 -> MinMax2/1
  MinMax5/1 -> Memory7/1, Add2/2

== system Twotanks_Model_TCGen/Anti-patternCalc7 ==
  OutSig : Inport
  Abs2 : Abs
  Abs3 : Abs
  Add1 : Sum  Inputs=+-
  Add2 : Sum  Inputs=+-
  Infinite1 : Scope
  Memory{3..7} (5 alike) : Memory
  MinMax2 : MinMax  Function=max  Inputs=2
  MinMax3 : MinMax  Function=max  Inputs=2
  MinMax4 : MinMax  Function=max  Inputs=2
  MinMax5 : MinMax  Inputs=2
  Rate Transition3 : RateTransition
  derive1 : Scope
  Infinite : Outport
  Derivative : Outport  Port=2
  MaxMin : Outport  Port=3
  wires:
  MinMax5/1 -> Add2/2, Memory7/1
  Abs2/1 -> MinMax2/1
  Memory4/1 -> MinMax3/2
  Memory3/1 -> MinMax2/2
  MinMax4/1 -> Add2/1, Memory6/1
  Memory7/1 -> MinMax5/2
  Add1/1 -> Abs2/1
  Memory6/1 -> MinMax4/2
  Memory5/1 -> Add1/2
  Rate Transition3/1 -> MinMax4/1, MinMax5/1, Abs3/1, Add1/1, Memory5/1
  Abs3/1 -> MinMax3/1
  MinMax2/1 -> Derivative/1, derive1/1, Memory3/1
  OutSig/1 -> Rate Transition3/1
  MinMax3/1 -> Memory4/1, Infinite/1, Infinite1/1
  Add2/1 -> MaxMin/1

== system Twotanks_Model_TCGen/Anti-patternCalc8 ==
  OutSig : Inport
  Abs2 : Abs
  Abs3 : Abs
  Add1 : Sum  Inputs=+-
  Add2 : Sum  Inputs=+-
  Infinite1 : Scope
  Memory{3..7} (5 alike) : Memory
  MinMax2 : MinMax  Function=max  Inputs=2
  MinMax3 : MinMax  Function=max  Inputs=2
  MinMax4 : MinMax  Function=max  Inputs=2
  MinMax5 : MinMax  Inputs=2
  Rate Transition3 : RateTransition
  derive1 : Scope
  Infinite : Outport
  Derivative : Outport  Port=2
  MaxMin : Outport  Port=3
  wires:
  MinMax5/1 -> Add2/2, Memory7/1
  Abs2/1 -> MinMax2/1
  Memory4/1 -> MinMax3/2
  Memory3/1 -> MinMax2/2
  MinMax4/1 -> Add2/1, Memory6/1
  Memory7/1 -> MinMax5/2
  Add1/1 -> Abs2/1
  Memory6/1 -> MinMax4/2
  Memory5/1 -> Add1/2
  Rate Transition3/1 -> MinMax4/1, MinMax5/1, Abs3/1, Add1/1, Memory5/1
  Abs3/1 -> MinMax3/1
  MinMax2/1 -> Derivative/1, derive1/1, Memory3/1
  OutSig/1 -> Rate Transition3/1
  MinMax3/1 -> Memory4/1, Infinite/1, Infinite1/1
  Add2/1 -> MaxMin/1

== system Twotanks_Model_TCGen/Anti-patternCalc9 ==
  OutSig : Inport
  Abs2 : Abs
  Abs3 : Abs
  Add1 : Sum  Inputs=+-
  Add2 : Sum  Inputs=+-
  Infinite1 : Scope
  Memory{3..7} (5 alike) : Memory
  MinMax2 : MinMax  Function=max  Inputs=2
  MinMax3 : MinMax  Function=max  Inputs=2
  MinMax4 : MinMax  Function=max  Inputs=2
  MinMax5 : MinMax  Inputs=2
  Rate Transition3 : RateTransition
  derive1 : Scope
  Infinite : Outport
  Derivative : Outport  Port=2
  MaxMin : Outport  Port=3
  wires:
  Add2/1 -> MaxMin/1
  MinMax3/1 -> Infinite1/1, Infinite/1, Memory4/1
  OutSig/1 -> Rate Transition3/1
  MinMax2/1 -> Memory3/1, derive1/1, Derivative/1
  Abs3/1 -> MinMax3/1
  Rate Transition3/1 -> Memory5/1, Add1/1, Abs3/1, MinMax5/1, MinMax4/1
  Memory5/1 -> Add1/2
  Memory6/1 -> MinMax4/2
  Add1/1 -> Abs2/1
  Memory7/1 -> MinMax5/2
  MinMax4/1 -> Memory6/1, Add2/1
  Memory3/1 -> MinMax2/2
  Memory4/1 -> MinMax3/2
  Abs2/1 -> MinMax2/1
  MinMax5/1 -> Memory7/1, Add2/2

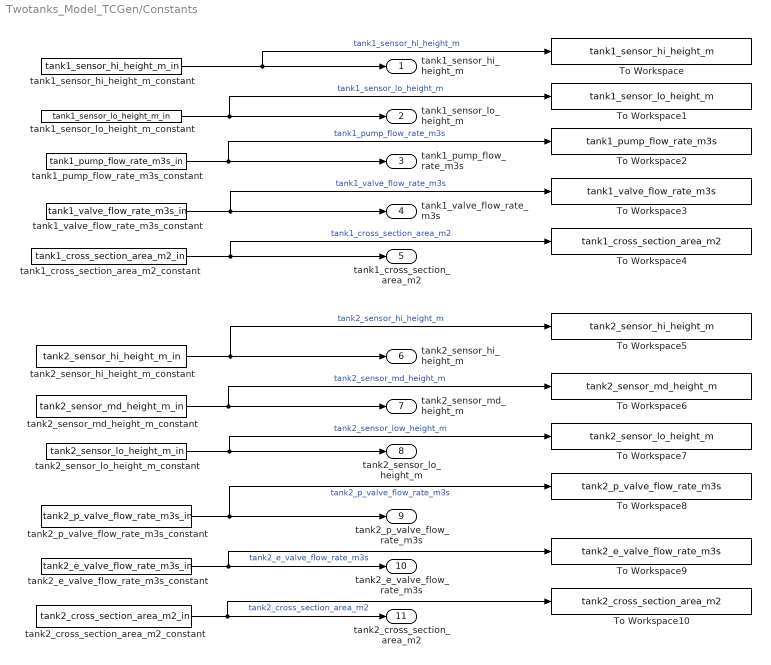
== system Twotanks_Model_TCGen/Constants ==
  To Workspace : ToWorkspace  VariableName=tank1_sensor_hi_height_m  SampleTime=-1
  To Workspace1 : ToWorkspace  VariableName=tank1_sensor_lo_height_m  SampleTime=-1
  To Workspace10 : ToWorkspace  VariableName=tank2_cross_section_area_m2  SampleTime=-1
  To Workspace2 : ToWorkspace  VariableName=tank1_pump_flow_rate_m3s  SampleTime=-1
  To Workspace3 : ToWorkspace  VariableName=tank1_valve_flow_rate_m3s  SampleTime=-1
  To Workspace4 : ToWorkspace  VariableName=tank1_cross_section_area_m2  SampleTime=-1
  To Workspace5 : ToWorkspace  VariableName=tank2_sensor_hi_height_m  SampleTime=-1
  To Workspace6 : ToWorkspace  VariableName=tank2_sensor_md_height_m  SampleTime=-1
  To Workspace7 : ToWorkspace  VariableName=tank2_sensor_lo_height_m  SampleTime=-1
  To Workspace8 : ToWorkspace  VariableName=tank2_p_valve_flow_rate_m3s  SampleTime=-1
  To Workspace9 : ToWorkspace  VariableName=tank2_e_valve_flow_rate_m3s  SampleTime=-1
  tank1_cross_section_area_m2_constant : Constant  Value=tank1_cross_section_area_m2_in
  tank1_pump_flow_rate_m3s_constant : Constant  Value=tank1_pump_flow_rate_m3s_in
  tank1_sensor_hi_height_m_constant : Constant  Value=tank1_sensor_hi_height_m_in
  tank1_sensor_lo_height_m_constant : Constant  Value=tank1_sensor_lo_height_m_in
  tank1_valve_flow_rate_m3s_constant : Constant  Value=tank1_valve_flow_rate_m3s_in
  tank2_cross_section_area_m2_constant : Constant  Value=tank2_cross_section_area_m2_in
  tank2_e_valve_flow_rate_m3s_constant : Constant  Value=tank2_e_valve_flow_rate_m3s_in
  tank2_p_valve_flow_rate_m3s_constant : Constant  Value=tank2_p_valve_flow_rate_m3s_in
  tank2_sensor_hi_height_m_constant : Constant  Value=tank2_sensor_hi_height_m_in
  tank2_sensor_lo_height_m_constant : Constant  Value=tank2_sensor_lo_height_m_in
  tank2_sensor_md_height_m_constant : Constant  Value=tank2_sensor_md_height_m_in
  tank1_sensor_hi_height_m : Outport
  tank1_sensor_lo_height_m : Outport  Port=2
  tank1_pump_flow_rate_m3s : Outport  Port=3
  tank1_valve_flow_rate_m3s : Outport  Port=4
  tank1_cross_section_area_m2 : Outport  Port=5
  tank2_sensor_hi_height_m : Outport  Port=6
  tank2_sensor_md_height_m : Outport  Port=7
  tank2_sensor_lo_height_m : Outport  Port=8
  tank2_p_valve_flow_rate_m3s : Outport  Port=9
  tank2_e_valve_flow_rate_m3s : Outport  Port=10
  tank2_cross_section_area_m2 : Outport  Port=11
  wires:
  tank2_sensor_hi_height_m_constant/1 -> To Workspace5/1, tank2_sensor_hi_height_m/1  "tank2_sensor_hi_height_m"
  tank2_sensor_lo_height_m_constant/1 -> To Workspace7/1, tank2_sensor_lo_height_m/1  "tank2_sensor_low_height_m"
  tank1_sensor_hi_height_m_constant/1 -> To Workspace/1, tank1_sensor_hi_height_m/1  "tank1_sensor_hi_height_m"
  tank1_pump_flow_rate_m3s_constant/1 -> tank1_pump_flow_rate_m3s/1, To Workspace2/1  "tank1_pump_flow_rate_m3s"
  tank1_cross_section_area_m2_constant/1 -> To Workspace4/1, tank1_cross_section_area_m2/1  "tank1_cross_section_area_m2"
  tank1_valve_flow_rate_m3s_constant/1 -> To Workspace3/1, tank1_valve_flow_rate_m3s/1  "tank1_valve_flow_rate_m3s"
  tank1_sensor_lo_height_m_constant/1 -> tank1_sensor_lo_height_m/1, To Workspace1/1  "tank1_sensor_lo_height_m"
  tank2_p_valve_flow_rate_m3s_constant/1 -> tank2_p_valve_flow_rate_m3s/1, To Workspace8/1  "tank2_p_valve_flow_rate_m3s"
  tank2_cross_section_area_m2_constant/1 -> To Workspace10/1, tank2_cross_section_area_m2/1  "tank2_cross_section_area_m2"
  tank2_e_valve_flow_rate_m3s_constant/1 -> To Workspace9/1, tank2_e_valve_flow_rate_m3s/1  "tank2_e_valve_flow_rate_m3s"
  tank2_sensor_md_height_m_constant/1 -> To Workspace6/1, tank2_sensor_md_height_m/1  "tank2_sensor_md_height_m"
